simulink model "exm2_6"  (Simulink 3.00)
settings: Solver=VariableStepDiscrete  SolverMode=SingleTasking  StartTime=0.0  StopTime=10.0  RelTol=1e-3  AbsTol=1e-6
settings Model: RTWTemplateMakefile=grt_vc.tmf

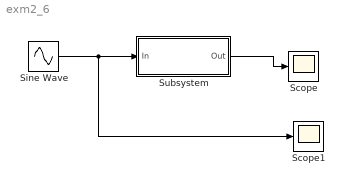
== system exm2_6 ==
  Scope : Scope
      settings: TickLabels=on  TimeRange=auto  YMin=-5  YMax=5  SaveToWorkspace=off  SaveName=ScopeData  DataFormat=Matrix
  Scope1 : Scope
      settings: TickLabels=on  TimeRange=auto  YMin=-5  YMax=5  SaveToWorkspace=off  SaveName=ScopeData  DataFormat=Matrix
  Sine Wave : Sin  Amplitude=1  Frequency=1  Phase=0  SampleTime=0
  Subsystem : Subsystem  mask(comparater){t=off}
      mask prompts: t "threshold on"
      mask help: The block will translate the input signal to square wave. If the checkbox 'threshold on' is selected then threshold is 0.5, otherwise, there is no threshold.
      mask init:
      | if t
      | th=0.5;
      | else
      | th=0;
      | end
      mask Help: Select the checkbox 'threshold on' to access the threshold function.
      mask Display: disp('The Comparater')
  wires:
  Subsystem/1(Out) -> Scope/1
  Sine Wave/1 -> Subsystem/1(In), Scope1/1

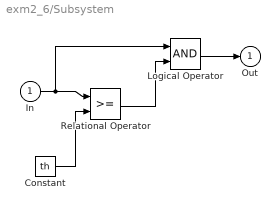
== system exm2_6/Subsystem ==
  In : Inport  Port=1  PortWidth=-1  SampleTime=-1  DataType=auto
      settings: SignalType=auto
  Constant : Constant  Value=th
  Logical Operator : Logic  Operator=AND  Inputs=2
  Relational Operator : RelationalOperator  Operator=>=
  Out : Outport  Port=1  InitialOutput=0
  wires:
  Relational Operator/1 -> Logical Operator/2
  Constant/1 -> Relational Operator/2
  In/1 -> Relational Operator/1, Logical Operator/1
  Logical Operator/1 -> Out/1
